simulink model "ProposedProblem1"  (R2013a)
settings: Solver=ode45  StartTime=0.0  StopTime=7200  RelTol=1e-3
undefined symbols (not defined in the file): des, gcbh
settings Model: Creator=gabig  LastModifiedBy=gabig

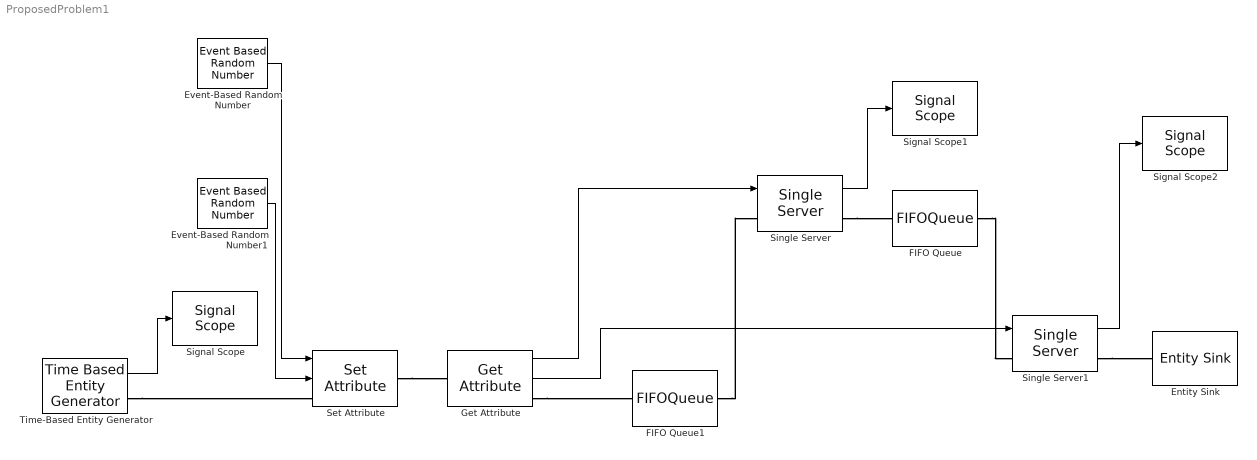
== system ProposedProblem1 ==
  Entity Sink : EntitySink
  Event-Based Random Number : EventBasedRandomNumber  Distribution=Uniform  minUnif=20  maxUnif=40  Seed=12348
  Event-Based Random Number1 : EventBasedRandomNumber  Distribution=Uniform  minUnif=120  maxUnif=240  Seed=12354
  FIFO Queue : FIFOQueue
  FIFO Queue1 : FIFOQueue
  Get Attribute : GetAttribute  AttributeName=ReadTime|Executetime  AttributeMissing=Error|Error  AttributeDefaultValue=1|1  AttributeTreatAsVector=1|1  AttributeSendTiming=After entity departure|After entity departure  EvaluatedDefaultAttributeValue={ [];[]}
      settings: OutputPortMap=o1,o2
  Set Attribute : SetAttribute  AttributeName=ReadTime|Executetime  AttributeFrom=Signal port|Signal port  AttributeValue=1|1  AttributeTreatAsVector=1|1  EvaluatedAttributeValue={ [];[]}
      settings: InputPortMap=u0,u1
  Signal Scope : SignalScope  LoadFcn=des.scope.CallbackSupport('seLoadFcn',gcbh)  StartFcn=des.scope.CallbackSupport('seStartFcn',gcbh)  StopFcn=des.scope.CallbackSupport('seStopFcn',gcbh)
      settings: CopyFcn=des.scope.CallbackSupport('seCopyFcn',gcbh)  DeleteFcn=des.scope.CallbackSupport('seDeleteFcn',gcbh)  PreSaveFcn=des.scope.CallbackSupport('sePreSaveFcn',gcbh)  NameChangeFcn=des.scope.CallbackSupport('seNameChangeFcn',gcbh)  OpenFcn=des.scope.CallbackSupport('seOpenFcn',gcbh)
  Signal Scope1 : SignalScope  LoadFcn=des.scope.CallbackSupport('seLoadFcn',gcbh)  StartFcn=des.scope.CallbackSupport('seStartFcn',gcbh)  StopFcn=des.scope.CallbackSupport('seStopFcn',gcbh)
      settings: CopyFcn=des.scope.CallbackSupport('seCopyFcn',gcbh)  DeleteFcn=des.scope.CallbackSupport('seDeleteFcn',gcbh)  PreSaveFcn=des.scope.CallbackSupport('sePreSaveFcn',gcbh)  NameChangeFcn=des.scope.CallbackSupport('seNameChangeFcn',gcbh)  OpenFcn=des.scope.CallbackSupport('seOpenFcn',gcbh)
  Signal Scope2 : SignalScope  LoadFcn=des.scope.CallbackSupport('seLoadFcn',gcbh)  StartFcn=des.scope.CallbackSupport('seStartFcn',gcbh)  StopFcn=des.scope.CallbackSupport('seStopFcn',gcbh)
      settings: CopyFcn=des.scope.CallbackSupport('seCopyFcn',gcbh)  DeleteFcn=des.scope.CallbackSupport('seDeleteFcn',gcbh)  PreSaveFcn=des.scope.CallbackSupport('sePreSaveFcn',gcbh)  NameChangeFcn=des.scope.CallbackSupport('seNameChangeFcn',gcbh)  OpenFcn=des.scope.CallbackSupport('seOpenFcn',gcbh)
  Single Server : SingleServer  ServiceTimeFrom=Signal port t  StatAverageWait=on
      settings: OutputPortMap=o4
  Single Server1 : SingleServer  ServiceTimeFrom=Signal port t  StatAverageWait=on
      settings: OutputPortMap=o4
  Time-Based Entity Generator : TimeBasedEntityGenerator  Distribution=Uniform  InitialSeed=12333  Minimum=60  Maximum=180  StatNumberDeparted=on
  wires:
  Event-Based Random Number1/1 -> Set Attribute/2
  Event-Based Random Number/1 -> Set Attribute/1
  Get Attribute/1 -> Single Server/1
  Get Attribute/2 -> Single Server1/1
  Time-Based Entity Generator/1 -> Signal Scope/1
  Single Server/1 -> Signal Scope1/1
  Single Server1/1 -> Signal Scope2/1
  connections:
  Single Server1/RConn1 -- Entity Sink/LConn1
  FIFO Queue1/RConn1 -- Single Server/LConn1
  Time-Based Entity Generator/RConn1 -- Set Attribute/LConn1
  Get Attribute/RConn1 -- FIFO Queue1/LConn1
  FIFO Queue/RConn1 -- Single Server1/LConn1
  Set Attribute/RConn1 -- Get Attribute/LConn1
  Single Server/RConn1 -- FIFO Queue/LConn1
